simulink subsystem "MotorSensor"  (R2025a)
settings: Solver=VariableStepAuto  StartTime=0.0  StopTime=10.0  RelTol=1e-3
libraries: fl_lib x4, nesl_utility x2
settings Model: Creator=upattacini  LastModifiedBy=upattacini
settings RTWCC: GPUComputeCapability=3.5

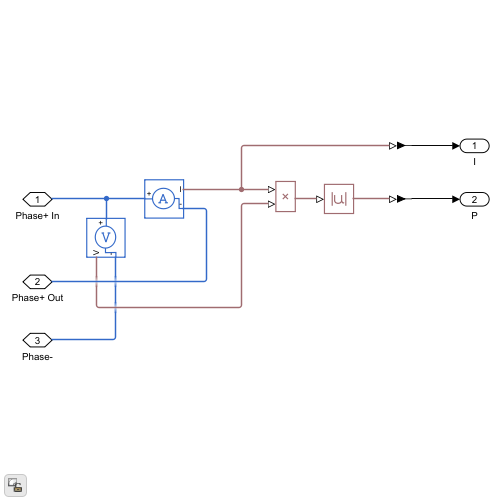
[thumbnail: Simulink's stored preview of the top-level diagram]
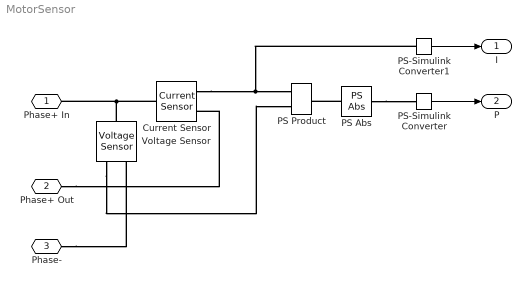
== system MotorSensor ==
  Current Sensor : fl_lib/Electrical/Electrical Sensors/Current Sensor
  PS Abs : fl_lib/Physical Signals/Nonlinear Operators/PS Abs  ZeroCross=true
      settings: InternalSimscapePortConfiguration="{\"Bottom\":[],\"Left\":[{\"id\":\"I\",\"label\":\"\",\"type\":\"input\"}],\"Right\":[{\"id\":\"O\",\"label\":\"\",\"type\":\"output\"}],\"Top\":[]}"
  PS Product : fl_lib/Physical Signals/Functions/PS Product
  PS-Simulink Converter : nesl_utility/PS-Simulink Converter  PhysicalDomain=network_engine_domain  SubClassName=ps_output  LeftPortType=input  RightPortType=output  PseudoPeriodic=off  Frequencies=[]  VectorFormat=inherit  Unit=W  AffineConversion=off
  PS-Simulink Converter1 : nesl_utility/PS-Simulink Converter  PhysicalDomain=network_engine_domain  SubClassName=ps_output  LeftPortType=input  RightPortType=output  PseudoPeriodic=off  Frequencies=[]  VectorFormat=inherit  Unit=A  AffineConversion=off
  Voltage Sensor : fl_lib/Electrical/Electrical Sensors/Voltage Sensor
  Phase+ In : PMIOPort  Side=Left
  Phase+ Out : PMIOPort  Port=2  Side=Left
  Phase- : PMIOPort  Port=3  Side=Left
  I : Outport
  P : Outport  Port=2
  wires:
  PS-Simulink Converter/1 -> P/1
  PS-Simulink Converter1/1 -> I/1
  connections:
  Current Sensor/RConn1 -- PS-Simulink Converter1/LConn1 -- PS Product/LConn1
  Voltage Sensor/LConn1 -- Current Sensor/LConn1 -- Phase+ In/RConn1
  PS Abs/RConn1 -- PS-Simulink Converter/LConn1
  PS Abs/LConn1 -- PS Product/RConn1
  Phase-/RConn1 -- Voltage Sensor/RConn2
  Voltage Sensor/RConn1 -- PS Product/LConn2
  Phase+ Out/RConn1 -- Current Sensor/RConn2
